simulink model "chap1_14"  (Simulink 3.00)
settings: Solver=ode45  StartTime=0.0  StopTime=4000  RelTol=1e-3
values from neighbouring files (symbols this model uses):
  kd = 0.01    [chap1_10.m]    (also in chap1_12.m = 10; chap1_13.m = 3; chap1_15.m = 0; chap1_16.m = 12)
  ki = 2.0    (= 2)    [chap1_10.m]    (also in chap1_12.m = 0.1; chap1_13.m = 0.005; chap1_15.m = 9; chap1_16.m = 0.0048)
  kp = 1.0    (= 1)    [chap1_10.m]    (also in chap1_12.m = 8; chap1_13.m = 0.8; chap1_15.m = 0.85; chap1_16.m = 0.45)
  ts = 0.001    [chap1_10.m]    (also in chap1_12.m; chap1_13.m = 20; chap1_15.m; chap1_16.m = 20)
undefined symbols (not defined in the file or in its folder): den, num

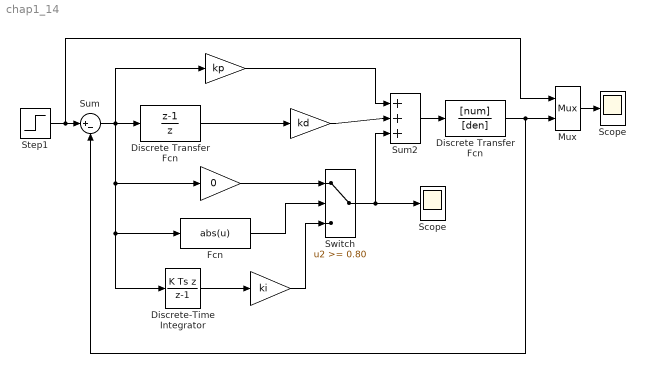
== system chap1_14 ==
  "  " : Gain  Gain=kp  SaturateOnIntegerOverflow=on
  "   " : Gain  Gain=ki  SaturateOnIntegerOverflow=on
  "    " : Gain  Gain=0  SaturateOnIntegerOverflow=on
  "     " : Gain  Gain=kd  SaturateOnIntegerOverflow=on
  Discrete Transfer Fcn : DiscreteTransferFcn  Numerator=[num]  Denominator=[den]  SampleTime=ts
  "Discrete Transfer Fcn " : DiscreteTransferFcn  Numerator=[1 -1]  Denominator=[1 0]  SampleTime=ts
  "Discrete-Time Integrator " : DiscreteIntegrator  IntegratorMethod=BackwardEuler  ExternalReset=none  InitialConditionSource=internal  InitialCondition=0  LimitOutput=off  UpperSaturationLimit=inf  LowerSaturationLimit=-inf  ShowSaturationPort=off  ShowStatePort=off  SampleTime=ts
  Fcn : Fcn  Expr=abs(u)
  Mux : Mux  Inputs=2
      settings: DisplayOption=none
  Scope : Scope
      settings: TimeRange=auto  YMin=1  YMax=1.00015  SaveToWorkspace=off  SaveName=ScopeData
  "Scope " : Scope
      settings: TimeRange=auto  YMin=-5  YMax=5  SaveToWorkspace=off  SaveName=ScopeData
  Step1 : Step  Time=0  Before=0  After=1  SampleTime=ts
  Sum : Sum  Inputs=|+-  SaturateOnIntegerOverflow=on
  Sum2 : Sum  Inputs=|+++  SaturateOnIntegerOverflow=on
  Switch : Switch  Threshold=0.80
  wires:
  "Discrete-Time Integrator "/1 -> "   "/1
  "    "/1 -> Switch/1
  Fcn/1 -> Switch/2
  "   "/1 -> Switch/3
  Mux/1 -> Scope/1
  Discrete Transfer Fcn/1 -> Sum/2, Mux/2
  "  "/1 -> Sum2/1
  Sum2/1 -> Discrete Transfer Fcn/1
  Switch/1 -> "Scope "/1, Sum2/3
  "     "/1 -> Sum2/2
  "Discrete Transfer Fcn "/1 -> "     "/1
  Step1/1 -> Sum/1, Mux/1
  Sum/1 -> "  "/1, "    "/1, "Discrete-Time Integrator "/1, Fcn/1, "Discrete Transfer Fcn "/1
